simulink model "Pendulum_Withm.FileR2020a"  (R2023b)
settings: Solver=VariableStepAuto  StartTime=0.0  StopTime=10.0  MaxStep=1e-3  RelTol=1e-3
values from neighbouring files (symbols this model uses):
  g = 9.81    [Pendulum.m]
  L = LenghtValue(i)    [Pendulum.m]
  th0 = 0.5    [Pendulum.m]
settings Model: Creator=hp  LastModifiedBy=hp

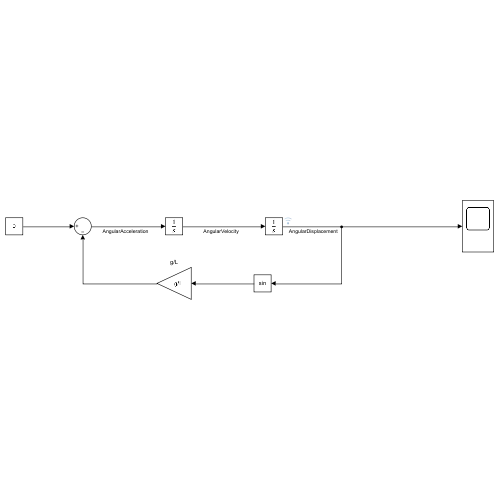
[thumbnail: Simulink's stored preview of the top-level diagram]
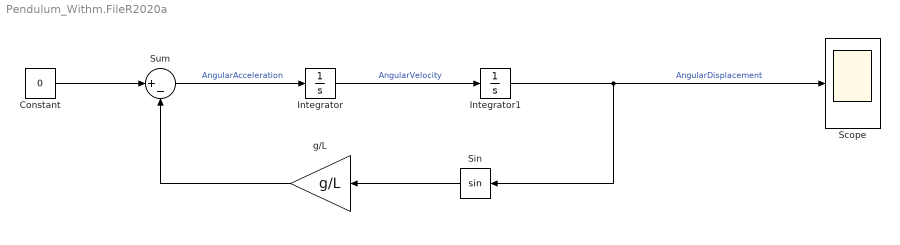
== system Pendulum_Withm.FileR2020a ==
  Constant : Constant  Value=0
  Integrator : Integrator
  Integrator1 : Integrator  InitialCondition=th0
  Scope : Scope
  Sin : Trigonometry
  Sum : Sum  Inputs=|+-
  g/L : Gain  Gain=g/L
  wires:
  Sin/1 -> g/L/1
  Integrator1/1 -> Scope/1, Sin/1  "AngularDisplacement"
  Integrator/1 -> Integrator1/1  "AngularVelocity"
  Sum/1 -> Integrator/1  "AngularAcceleration"
  Constant/1 -> Sum/1
  g/L/1 -> Sum/2
